simulink model "Experiment_TF"  (R2023b)
settings: Solver=VariableStepAuto  StartTime=0.0  StopTime=10  RelTol=1e-5
values from neighbouring files (symbols this model uses):
  C_DEN = C_DEN{1}    [WOK.m]    (also in systune.m = tf(controllerSysTuned).Denominator{1})
  C_NUM = C_NUM{1}    [WOK.m]    (also in systune.m = tf(controllerSysTuned).Numerator{1})
  G = ballOnBeam()    [WOK.m]    (also in looptune.m = plantSys; systune.m = ss(plantSys))
  GX0 = zeros(Cdim(2), 1)    [WOK.m]    (also in systune.m)
libraries: dspsrcs4 x4
settings Model: Creator=Alex  LastModifiedBy=Alex

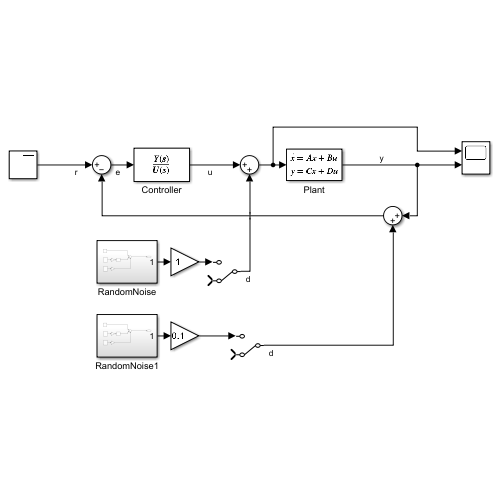
[thumbnail: Simulink's stored preview of the top-level diagram]
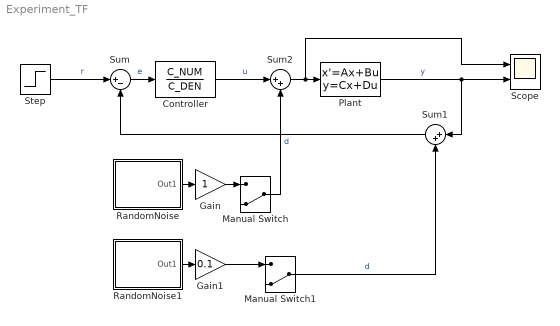
== system Experiment_TF ==
  Controller : TransferFcn  Numerator=C_NUM  Denominator=C_DEN
  Gain : Gain
  Gain1 : Gain  Gain=0.1
  Manual Switch : ManualSwitch  CurrentSetting=0
  Manual Switch1 : ManualSwitch  CurrentSetting=0
  Plant : StateSpace  A=G.A  B=G.B  C=G.C  D=G.D  InitialCondition=GX0  AllowTunableDMatrix=on  ContinuousStateAttributes='state'
  RandomNoise : Subsystem
  RandomNoise1 : Subsystem
  Scope : Scope  NumInputPorts=2
  Step : Step  Time=0.1  SampleTime=0
  Sum : Sum  Inputs=|+-
  Sum1 : Sum  Inputs=|++
  Sum2 : Sum  Inputs=|++
  wires:
  Step/1 -> Sum/1  "r"
  Sum/1 -> Controller/1  "e"
  Plant/1 -> Sum1/1, Scope/2  "y"
  Controller/1 -> Sum2/1  "u"
  Sum2/1 -> Scope/1, Plant/1
  Manual Switch/1 -> Sum2/2  "d"
  RandomNoise/1(Out1) -> Gain/1
  Sum1/1 -> Sum/2
  Manual Switch1/1 -> Sum1/2  "d"
  Gain/1 -> Manual Switch/1
  RandomNoise1/1(Out1) -> Gain1/1
  Gain1/1 -> Manual Switch1/1

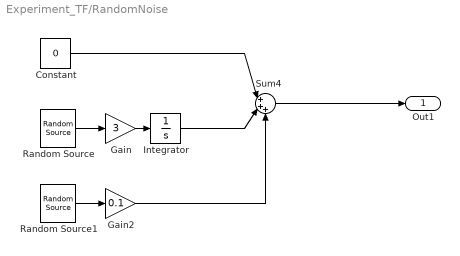
== system Experiment_TF/RandomNoise ==
  Constant : Constant  Value=0
  Gain : Gain  Gain=3
  Gain2 : Gain  Gain=0.1
  Integrator : Integrator
  Random Source : dspsrcs4/Random Source  SrcType=Uniform  NormMethod=Ziggurat  CltLength=12  MinVal=-1  MaxVal=1  MeanVal=0  VarVal=1  RepMode=Not repeatable  rawSeed=1  IsInherit=off  SampMode=Discrete  SampTime=0.1  SampFrame=1  DataType=Double  OutComplex=Real  OutputFrames=off
  Random Source1 : dspsrcs4/Random Source  SrcType=Uniform  NormMethod=Ziggurat  CltLength=12  MinVal=-1  MaxVal=1  MeanVal=0  VarVal=1  RepMode=Not repeatable  rawSeed=1  IsInherit=off  SampMode=Discrete  SampTime=0.05  SampFrame=1  DataType=Double  OutComplex=Real  OutputFrames=off
  Sum4 : Sum  Inputs=|+++
  Out1 : Outport
  wires:
  Sum4/1 -> Out1/1
  Gain/1 -> Integrator/1
  Random Source/1 -> Gain/1
  Gain2/1 -> Sum4/3
  Random Source1/1 -> Gain2/1
  Integrator/1 -> Sum4/2
  Constant/1 -> Sum4/1

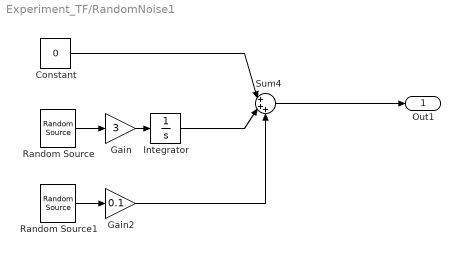
== system Experiment_TF/RandomNoise1 ==
  Constant : Constant  Value=0
  Gain : Gain  Gain=3
  Gain2 : Gain  Gain=0.1
  Integrator : Integrator
  Random Source : dspsrcs4/Random Source  SrcType=Uniform  NormMethod=Ziggurat  CltLength=12  MinVal=-1  MaxVal=1  MeanVal=0  VarVal=1  RepMode=Not repeatable  rawSeed=1  IsInherit=off  SampMode=Discrete  SampTime=0.1  SampFrame=1  DataType=Double  OutComplex=Real  OutputFrames=off
  Random Source1 : dspsrcs4/Random Source  SrcType=Uniform  NormMethod=Ziggurat  CltLength=12  MinVal=-1  MaxVal=1  MeanVal=0  VarVal=1  RepMode=Not repeatable  rawSeed=1  IsInherit=off  SampMode=Discrete  SampTime=0.05  SampFrame=1  DataType=Double  OutComplex=Real  OutputFrames=off
  Sum4 : Sum  Inputs=|+++
  Out1 : Outport
  wires:
  Sum4/1 -> Out1/1
  Gain/1 -> Integrator/1
  Random Source/1 -> Gain/1
  Gain2/1 -> Sum4/3
  Random Source1/1 -> Gain2/1
  Integrator/1 -> Sum4/2
  Constant/1 -> Sum4/1
